simulink model "ControlloDigitale_PosizionePendolo"  (R2023a)
settings: Solver=VariableStepAuto  StartTime=0.0  StopTime=t_f  MaxStep=MaxStep  RelTol=RelTol
values from neighbouring files (symbols this model uses):
  A_alpha = I + Ts*(I - alpha*A_ctrl*Ts)^-1*A_ctrl    [p89_ControlloDigitale_PosizionePendolo.m]
  b = 0.1    [p89_ControlloDigitale_PosizionePendolo.m]
  B_alpha_1 = (1 - alpha)*Ts*(I - alpha*A_ctrl*Ts)^-1*B_ctrl    [p89_ControlloDigitale_PosizionePendolo.m]
  B_alpha_2 = alpha*Ts*(I - alpha*A_ctrl*Ts)^-1*B_ctrl    [p89_ControlloDigitale_PosizionePendolo.m]
  C_ctrl = R_lti.C    [p89_ControlloDigitale_PosizionePendolo.m]
  C_star = M*g*l*sin(theta_star)    [p89_ControlloDigitale_PosizionePendolo.m]
  D_ctrl = R_lti.D    [p89_ControlloDigitale_PosizionePendolo.m]
  g = 9.81    [p89_ControlloDigitale_PosizionePendolo.m]
  k_inner = 0.79    [p89_ControlloDigitale_PosizionePendolo.m]
  l = 0.3    [p89_ControlloDigitale_PosizionePendolo.m]
  M = 0.5    [p89_ControlloDigitale_PosizionePendolo.m]
  theta_star = 2*pi/3    (= 2.09439510239)    [p89_ControlloDigitale_PosizionePendolo.m]
  Ts = 0.03    [p89_ControlloDigitale_PosizionePendolo.m]
settings Model: Creator=alessandro  LastModifiedBy=admin
settings OptimizationCC: ReuseModelBlockBuffer=off

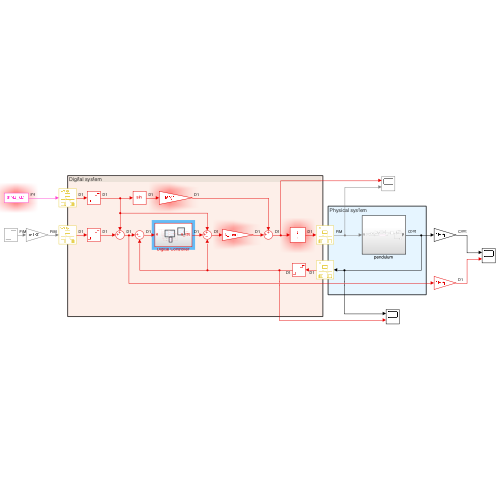
[thumbnail: Simulink's stored preview of the top-level diagram]
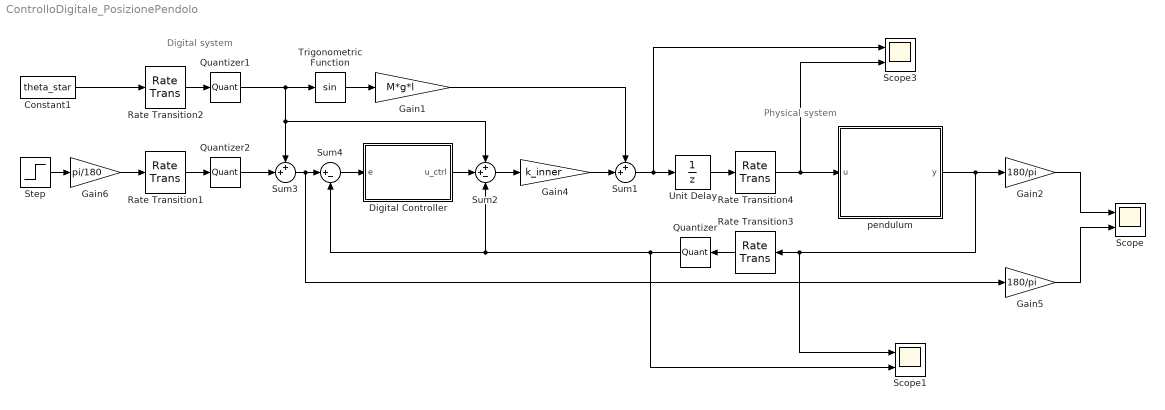
== system ControlloDigitale_PosizionePendolo ==
  note: Digital system
  note: Physical system
  Constant1 : Constant  Value=theta_star
  Digital Controller : Subsystem
  Gain1 : Gain  Gain=M*g*l
  Gain2 : Gain  Gain=180/pi
  Gain4 : Gain  Gain=k_inner
  Gain5 : Gain  Gain=180/pi
  Gain6 : Gain  Gain=pi/180
  Quantizer : Quantizer  QuantizationInterval=2*pi/2^15
  Quantizer1 : Quantizer  QuantizationInterval=2*pi/2^15
  Quantizer2 : Quantizer  QuantizationInterval=2*pi/2^15
  Rate Transition1 : RateTransition  Integrity=off  OutPortSampleTime=Ts
  Rate Transition2 : RateTransition  Integrity=off  OutPortSampleTime=Ts
  Rate Transition3 : RateTransition  Integrity=off  OutPortSampleTime=Ts
  Rate Transition4 : RateTransition  Integrity=off  OutPortSampleTime=0
  Scope : Scope  NumInputPorts=2
  Scope1 : Scope  NumInputPorts=2
  Scope3 : Scope  NumInputPorts=2
  Step : Step  SampleTime=0
  Sum1 : Sum  Inputs=++|
  Sum2 : Sum  Inputs=++-
  Sum3 : Sum  Inputs=++|
  Sum4 : Sum  Inputs=|+-
  Trigonometric Function : Trigonometry
  Unit Delay : UnitDelay  InitialCondition=C_star  SampleTime=Ts  HasFrameUpgradeWarning=on
  pendulum : Subsystem
  wires:
  Sum2/1 -> Gain4/1
  Gain4/1 -> Sum1/2
  Gain1/1 -> Sum1/1
  Trigonometric Function/1 -> Gain1/1
  Sum1/1 -> Unit Delay/1, Scope3/1
  pendulum/1(y) -> Gain2/1, Scope1/1, Rate Transition3/1
  Constant1/1 -> Rate Transition2/1
  Digital Controller/1(u_ctrl) -> Sum2/2
  Sum3/1 -> Gain5/1, Sum4/1
  Gain2/1 -> Scope/1
  Gain5/1 -> Scope/2
  Gain6/1 -> Rate Transition1/1
  Step/1 -> Gain6/1
  Rate Transition3/1 -> Quantizer/1
  Rate Transition1/1 -> Quantizer2/1
  Rate Transition2/1 -> Quantizer1/1
  Rate Transition4/1 -> pendulum/1(u), Scope3/2
  Sum4/1 -> Digital Controller/1(e)
  Unit Delay/1 -> Rate Transition4/1
  Quantizer/1 -> Scope1/2, Sum2/3, Sum4/2
  Quantizer1/1 -> Trigonometric Function/1, Sum2/1, Sum3/1
  Quantizer2/1 -> Sum3/2

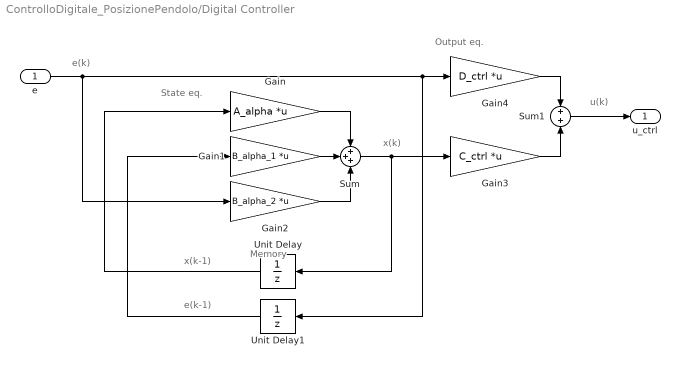
== system ControlloDigitale_PosizionePendolo/Digital Controller ==
  note: Memory
  note: e(k)
  note: x(k)
  note: x(k-1)
  note: e(k-1)
  note: u(k)
  note: State eq.
  note: Output eq.
  e : Inport
  Gain : Gain  Gain=A_alpha  Multiplication=Matrix(K*u)
  Gain1 : Gain  Gain=B_alpha_1  Multiplication=Matrix(K*u)
  Gain2 : Gain  Gain=B_alpha_2  Multiplication=Matrix(K*u)
  Gain3 : Gain  Gain=C_ctrl  Multiplication=Matrix(K*u)
  Gain4 : Gain  Gain=D_ctrl  Multiplication=Matrix(K*u)
  Sum : Sum  Inputs=+++
  Sum1 : Sum
  Unit Delay : UnitDelay  SampleTime=Ts  HasFrameUpgradeWarning=on
  Unit Delay1 : UnitDelay  SampleTime=Ts  HasFrameUpgradeWarning=on
  u_ctrl : Outport
  wires:
  e/1 -> Gain4/1, Unit Delay1/1, Gain2/1
  Unit Delay/1 -> Gain/1
  Unit Delay1/1 -> Gain1/1
  Gain1/1 -> Sum/2
  Gain/1 -> Sum/1
  Gain2/1 -> Sum/3
  Sum/1 -> Unit Delay/1, Gain3/1
  Gain4/1 -> Sum1/1
  Gain3/1 -> Sum1/2
  Sum1/1 -> u_ctrl/1

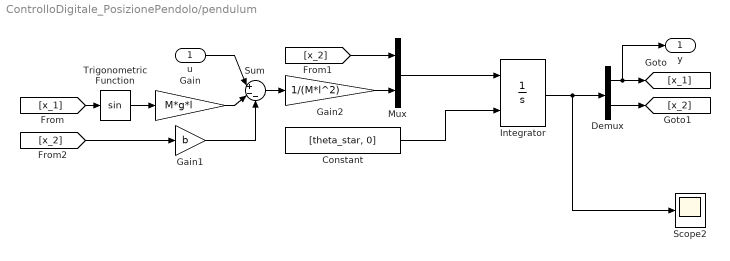
== system ControlloDigitale_PosizionePendolo/pendulum ==
  u : Inport
  Constant : Constant  Value=[theta_star, 0]
  Demux : Demux  Outputs=2
  Gain : Gain  Gain=M*g*l
  Gain1 : Gain  Gain=b
  Gain2 : Gain  Gain=1/(M*l^2)
  Integrator : Integrator  InitialConditionSource=external
  Mux : Mux  Inputs=2
  Scope2 : Scope
  Sum : Sum  Inputs=|+--
  Trigonometric Function : Trigonometry
  y : Outport
  wires:
  [x_2] -> Gain1/1
  Mux/1 -> Integrator/1
  Sum/1 -> Gain2/1
  Demux/2 -> [x_2]
  Integrator/1 -> Scope2/1, Demux/1
  Demux/1 -> y/1, [x_1]
  Gain1/1 -> Sum/3
  Gain2/1 -> Mux/2
  [x_1] -> Trigonometric Function/1
  Constant/1 -> Integrator/2
  Gain/1 -> Sum/2
  Trigonometric Function/1 -> Gain/1
  [x_2] -> Mux/1
  u/1 -> Sum/1
